simulink model "mohinh"  (R2017a)
settings: Solver=FixedStepDiscrete  StartTime=0.0  StopTime=5  RelTol=1e-3
undefined symbols (not defined in the file): ln
libraries: powerlib x16, electricdrivelib x2, simulink x1, re_lib x1
settings Model: Creator=huynh_000  LastModifiedBy=huynh_000

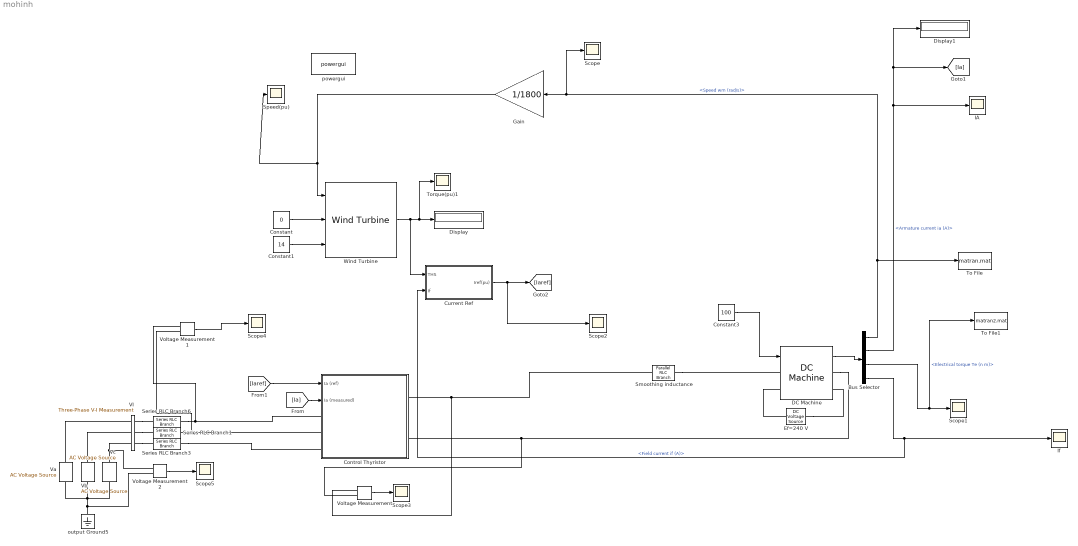
== system mohinh ==
  Bus Selector : BusSelector  OutputSignals=Speed wm (rad/s),Armature current ia (A),Electrical torque Te (n m),Field current if (A)
  Constant : Constant  Value=0
  Constant1 : Constant  Value=14
  Constant3 : Constant  Value=100
  Control Thyristor : Subsystem
  Current Ref : Subsystem
  DC Machine : powerlib/Machines/DC Machine  PresetModel=No  MechanicalLoad=Torque TL  FieldType=Wound  ShowDetailedParameters=on  MeasurementBus=off  RLa="[ 0.5  0.01]"  RLf="[240  120]"  Laf=1.8  MachineConstant=Torque constant (N.m/A)  Ke=1.8  Kt=1.8  J=2  Bm=0.5  Tf=0  w0=1  Ifinit=1  TsPowergui=0  TsBlock=-1
  Display : Display
  Display1 : Display
  Ef=240 V : powerlib/Electrical Sources/DC Voltage Source  Description=source block  Amplitude=240  Measurements=None
      settings: AttributesFormatString=\n
  Gain : Gain  Gain=1/1800
  IA : Scope
  If : Scope
  Scope{,1..5} (6 alike) : Scope
  Series RLC Branch1 : powerlib/Elements/Series RLC Branch  LConnTagsString=__new0  RConnTagsString=__new0  BranchType=RL  Resistance=0.01  Inductance=1e-3  SetiL0=off  InitialCurrent=0  Capacitance=[]  Setx0=off  InitialVoltage=0  Measurements=None
  Series RLC Branch3 : powerlib/Elements/Series RLC Branch  LConnTagsString=__new0  RConnTagsString=__new0  BranchType=RL  Resistance=0.01  Inductance=1e-3  SetiL0=off  InitialCurrent=0  Capacitance=[]  Setx0=off  InitialVoltage=0  Measurements=None
  Series RLC Branch6 : powerlib/Elements/Series RLC Branch  LConnTagsString=__new0  RConnTagsString=__new0  BranchType=RL  Resistance=0.01  Inductance=1e-3  SetiL0=off  InitialCurrent=0  Capacitance=[]  Setx0=off  InitialVoltage=0  Measurements=None
  Smoothing inductance : powerlib/Elements/Parallel RLC Branch  LConnTagsString=a  RConnTagsString=__new0  BranchType=L  Resistance=[]  Inductance=50e-3  SetiL0=off  InitialCurrent=0  Capacitance=[]  Setx0=off  InitialVoltage=0  Measurements=None
  Speed(pu) : Scope
  To File : ToFile  Filename=matran.mat  MatrixName=speed
  To File1 : ToFile  Filename=matran2.mat  MatrixName=torque
  Torque(pu)1 : Scope
  VI : powerlib/Measurements/Three-Phase V-I Measurement  VoltageMeasurement=phase-to-ground  SetLabelV=on  LabelV=Vabc  Vpu=on  VpuLL=off  CurrentMeasurement=yes  SetLabelI=on  LabelI=Iabc  Ipu=off  Pbase=100e6  Vbase=208  OutputType=Complex  PhasorSimulation=off  PSBequivalent=0
  Va : powerlib/Electrical Sources/AC Voltage Source  Description=source block  Amplitude=220*sqrt(2)  Phase=0  Frequency=60  SampleTime=0  Measurements=None  BusType=swing  Pref=10e3  Qref=0  Qmin=-inf  Qmax=+inf
      settings: AttributesFormatString=\n
  Vb : powerlib/Electrical Sources/AC Voltage Source  Description=source block  Amplitude=220*sqrt(2)  Phase=-120  Frequency=60  SampleTime=0  Measurements=None  BusType=swing  Pref=10e3  Qref=0  Qmin=-inf  Qmax=+inf
      settings: AttributesFormatString=\n
  Vc : powerlib/Electrical Sources/AC Voltage Source  Description=source block  Amplitude=220*sqrt(2)  Phase=120  Frequency=60  SampleTime=0  Measurements=None  BusType=swing  Pref=10e3  Qref=0  Qmin=-inf  Qmax=+inf
      settings: AttributesFormatString=\n
  Voltage Measurement : powerlib/Measurements/Voltage Measurement  PhasorSimulation=off  OutputType=Complex  PSBequivalent=0
  Voltage Measurement1 : powerlib/Measurements/Voltage Measurement  PhasorSimulation=off  OutputType=Complex  PSBequivalent=0
  Voltage Measurement2 : powerlib/Measurements/Voltage Measurement  PhasorSimulation=off  OutputType=Complex  PSBequivalent=0
  Wind Turbine : re_lib/Wind Generation/Wind Turbine  Pnom=20000  Pelec_base=20000/0.9  wind_base=12  P_wind_base=0.73  speed_nom=1.2  pitch_angle=0  c1_c6="[0.51763          116          0.4            5           21     0.006795]"  cp_nom=0.48  lambda_nom=8.1
      settings: SourceProductName=Simscape Power Systems  SourceProductBaseCode=PS
  output Ground5 : powerlib/Elements/Ground  LConnTagsString=a
  powergui : powerlib/powergui  Priority=1  SimulationMode=Discrete  SampleTime=0.001  frequency=60  Iterations=50  frequencyindice=0  Pbase=100e6  ErrMax=1e-4  UnitsV=kV  UnitsW=MW  buscounter=0  FunctionMessages=off  echomessages=off  EnableUseOfTLC=off  CurrentSourceSwitches=off  DisableSnubberDevices=off  DisableRonSwitches=off  DisableVfSwitches=off  DisplayEquations=off  SolverType=Tustin/Backward Euler (TBE)  Interpol=off  ExternalGateDelay=off  methode=off  Ts=100  x0status=blocks  SPID=on  SwTol=0  HookPort=off  RestoreLinks=warning  ResistiveCurrentMeasurement=off  Frange=[0:2:500]  Ylog=off  Xlog=on  ShowGrid=off  save=off  variable=ZData  structure=0  ZoomFFT=off  StartTime=0.0  cycles=1  DisplayStyle=1  fundamental=60  FreqAxis=off  MaxFrequency=1000  frequencyindicesteady=1  RmsSteady=1  display=off
  wires:
  Constant/1 -> Wind Turbine/2
  Constant1/1 -> Wind Turbine/3
  DC Machine/1 -> Bus Selector/1
  Bus Selector/1 -> To File/1, Scope/1, Gain/1  "<Speed wm (rad/s)>"
  Bus Selector/2 -> Display1/1, [Ia], IA/1  "<Armature current ia (A)>"
  [Ia] -> Control Thyristor/2("Ia (measured) ")
  Wind Turbine/1 -> Current Ref/1(THS), Torque(pu)1/1, Display/1
  Current Ref/1(Iref(pu)) -> Scope2/1, [Iaref]
  [Iaref] -> Control Thyristor/1("Ia (ref) ")
  Gain/1 -> Speed(pu)/1, Wind Turbine/1
  Bus Selector/3 -> To File1/1, Scope1/1  "<Electrical torque Te (n m)>"
  Bus Selector/4 -> Current Ref/2(If), If/1  "<Field current if (A)>"
  Voltage Measurement/1 -> Scope3/1
  Voltage Measurement1/1 -> Scope4/1
  Constant3/1 -> DC Machine/1
  Voltage Measurement2/1 -> Scope5/1
  connections:
  Series RLC Branch6/RConn1 -- Voltage Measurement1/LConn1 -- Control Thyristor/LConn1
  Smoothing inductance/RConn1 -- DC Machine/LConn1
  Smoothing inductance/LConn1 -- Voltage Measurement/LConn1 -- Control Thyristor/RConn1
  DC Machine/RConn1 -- Voltage Measurement/LConn2 -- Control Thyristor/RConn2
  Ef=240 V/RConn1 -- DC Machine/LConn2
  Ef=240 V/LConn1 -- DC Machine/RConn2
  Vb/LConn1 -- Voltage Measurement2/LConn2 -- output Ground5/LConn1 -- Vc/LConn1 -- Va/LConn1
  VI/RConn2 -- Series RLC Branch1/LConn1
  Vb/RConn1 -- VI/LConn2
  Va/RConn1 -- VI/LConn1
  VI/RConn3 -- Series RLC Branch3/LConn1
  Vc/RConn1 -- Voltage Measurement2/LConn1 -- VI/LConn3
  VI/RConn1 -- Series RLC Branch6/LConn1
  Series RLC Branch3/RConn1 -- Control Thyristor/LConn3
  Series RLC Branch1/RConn1 -- Voltage Measurement1/LConn2 -- Control Thyristor/LConn2

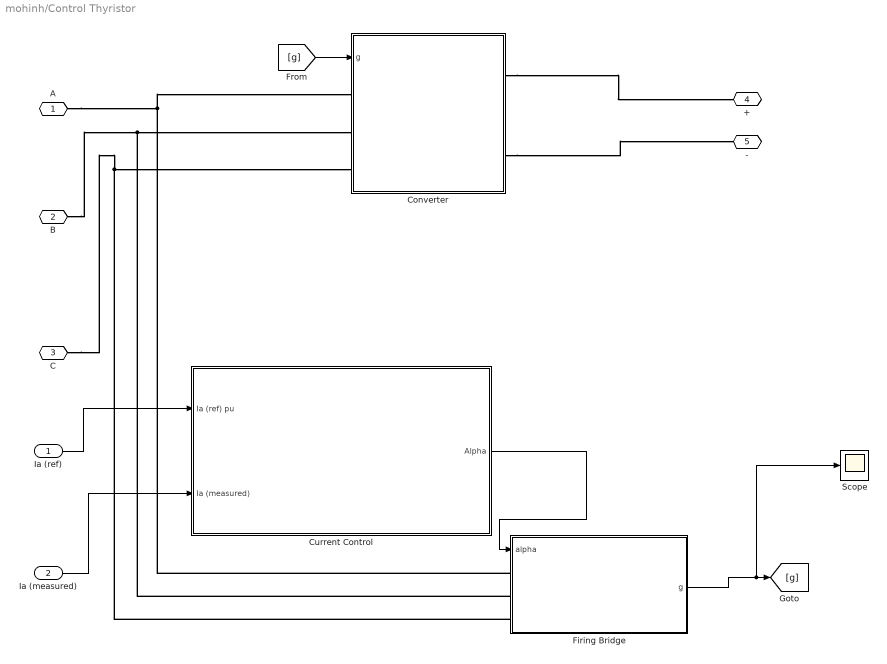
== system mohinh/Control Thyristor ==
  "Ia (ref) " : Inport
  "Ia (measured) " : Inport  Port=2
  Converter : Subsystem
  Current Control : Subsystem
  Firing Bridge : Subsystem
  Scope : Scope
  A : PMIOPort  Port=1  Side=Left
  B : PMIOPort  Port=2  Side=Left
  C : PMIOPort  Port=3  Side=Left
  + : PMIOPort  Tag=PMCPort  Port=4  Side=Right
  - : PMIOPort  Tag=PMCPort  Port=5  Side=Right
  wires:
  [g] -> Converter/1("g ")
  Firing Bridge/1("g ") -> Scope/1, [g]
  Current Control/1(" Alpha") -> Firing Bridge/1(alpha)
  "Ia (ref) "/1 -> Current Control/1(Ia (ref) pu)
  "Ia (measured) "/1 -> Current Control/2(Ia (measured))
  connections:
  A/RConn1 -- Firing Bridge/LConn1 -- Converter/LConn1
  B/RConn1 -- Firing Bridge/LConn2 -- Converter/LConn2
  C/RConn1 -- Firing Bridge/LConn3 -- Converter/LConn3
  Converter/RConn1 -- +/RConn1
  Converter/RConn2 -- -/RConn1

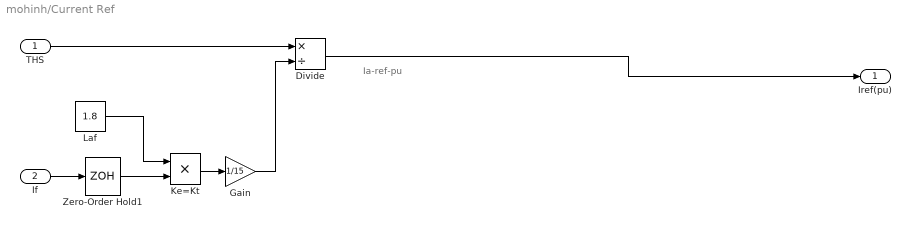
== system mohinh/Current Ref ==
  note: Ia-ref-pu
  THS : Inport
  If : Inport  Port=2
  Divide : Product  Inputs=*/
  Gain : Gain  Gain=1/15
  Ke=Kt : Product
  Laf : Constant  Value=1.8
  Zero-Order Hold1 : ZeroOrderHold  SampleTime=-1
  Iref(pu) : Outport
  wires:
  Laf/1 -> Ke=Kt/1
  THS/1 -> Divide/1
  If/1 -> Zero-Order Hold1/1
  Zero-Order Hold1/1 -> Ke=Kt/2
  Ke=Kt/1 -> Gain/1
  Gain/1 -> Divide/2
  Divide/1 -> Iref(pu)/1

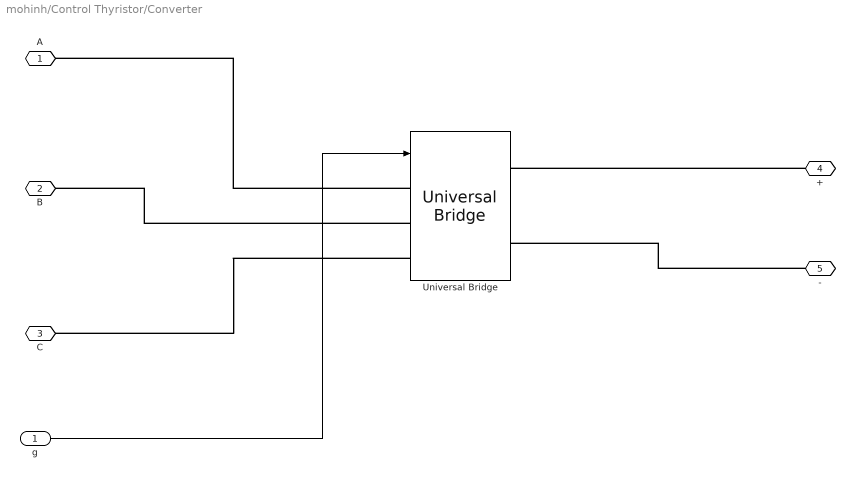
== system mohinh/Control Thyristor/Converter ==
  "g " : Inport
  Universal Bridge : powerlib/Power Electronics/Universal Bridge  Arms=3  SnubberResistance=1e5  SnubberCapacitance=inf  Device=Thyristors  Ron=1e-3  Lon=0  ForwardVoltages="[  0  0  ]"  ForwardVoltage=0  GTOparameters=[ 10e-6 , 20e-6 ]  IGBTparameters=[ 1e-6 , 2e-6 ]  Measurements=None  Measurements_2=None  converterType=Rectifier
  A : PMIOPort  Port=1  Side=Left
  B : PMIOPort  Port=2  Side=Left
  C : PMIOPort  Port=3  Side=Left
  + : PMIOPort  Tag=PMCPort  Port=4  Side=Right
  - : PMIOPort  Tag=PMCPort  Port=5  Side=Right
  wires:
  "g "/1 -> Universal Bridge/1
  connections:
  Universal Bridge/LConn1 -- A/RConn1
  Universal Bridge/LConn2 -- B/RConn1
  Universal Bridge/LConn3 -- C/RConn1
  +/RConn1 -- Universal Bridge/RConn1
  -/RConn1 -- Universal Bridge/RConn2

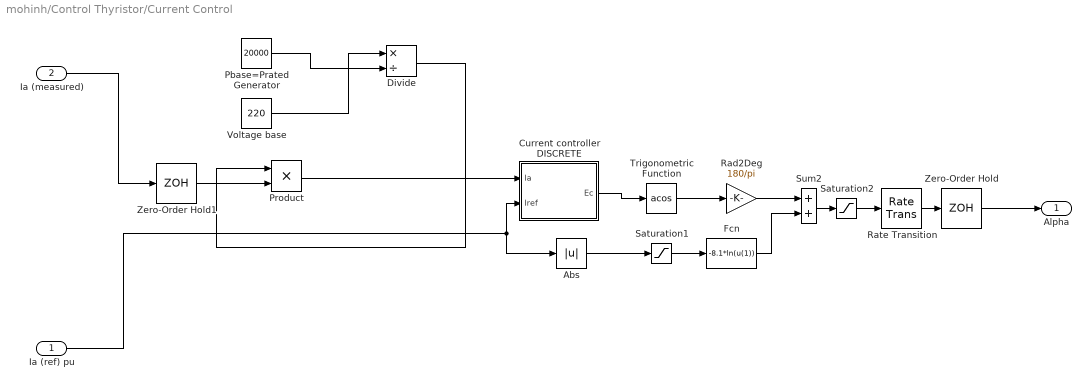
== system mohinh/Control Thyristor/Current Control ==
  Ia (ref) pu : Inport
  Ia (measured) : Inport  Port=2
  Abs : Abs  SaturateOnIntegerOverflow=on
  Current controller DISCRETE : Subsystem  AncestorBlock=|  mask(PI controller){Kp=1, Ki=80, Ts=100e-6}
      | electricdrivelib/Fundamental Drive Blocks/Current Controller
      | (DC)/current_controller/Rectifier_2q/Current controller
      | DISCRETE
      mask prompts: Kp "Proportional gain (Kp)"; Ki "Integral gain (Ki)"; Ts "Sample time (s) :"
      mask help: Proportional-Integral Speed Controller
      mask Display: plot(0,0,100,100,[35,35,65],[70,30,30],[35,65],[45,60])
  Divide : Product  Inputs=*/
  Fcn : Fcn  Expr=-8.1*ln(u(1))
  Pbase=Prated Generator : Constant  Value=20000
  Product : Product
  Rad2Deg : Gain  Gain=180/pi  SaturateOnIntegerOverflow=on  OutDataTypeStr=Inherit: Same as input  ParamDataTypeStr=Inherit: Same as input
  Rate Transition : RateTransition
  Saturation1 : Saturate  UpperLimit=1  LowerLimit=0.0005
  Saturation2 : Saturate  UpperLimit=160  LowerLimit=20
  Sum2 : Sum  SaturateOnIntegerOverflow=on  InputSameDT=on  OutDataTypeStr=Inherit: Same as first input
  Trigonometric Function : Trigonometry  Operator=acos
  Voltage base : Constant  Value=220
  Zero-Order Hold : ZeroOrderHold  SampleTime=100e-6
  Zero-Order Hold1 : ZeroOrderHold  SampleTime=100e-6
  " Alpha" : Outport
  wires:
  Saturation1/1 -> Fcn/1
  Abs/1 -> Saturation1/1
  Rad2Deg/1 -> Sum2/1
  Trigonometric Function/1 -> Rad2Deg/1
  Fcn/1 -> Sum2/2
  Ia (measured)/1 -> Zero-Order Hold1/1
  Zero-Order Hold/1 -> " Alpha"/1
  Saturation2/1 -> Rate Transition/1
  Product/1 -> Current controller DISCRETE/1(Ia)
  Ia (ref) pu/1 -> Current controller DISCRETE/2(Iref), Abs/1
  Current controller DISCRETE/1(Ec) -> Trigonometric Function/1
  Rate Transition/1 -> Zero-Order Hold/1
  Sum2/1 -> Saturation2/1
  Zero-Order Hold1/1 -> Product/2
  Voltage base/1 -> Divide/1
  Pbase=Prated Generator/1 -> Divide/2
  Divide/1 -> Product/1

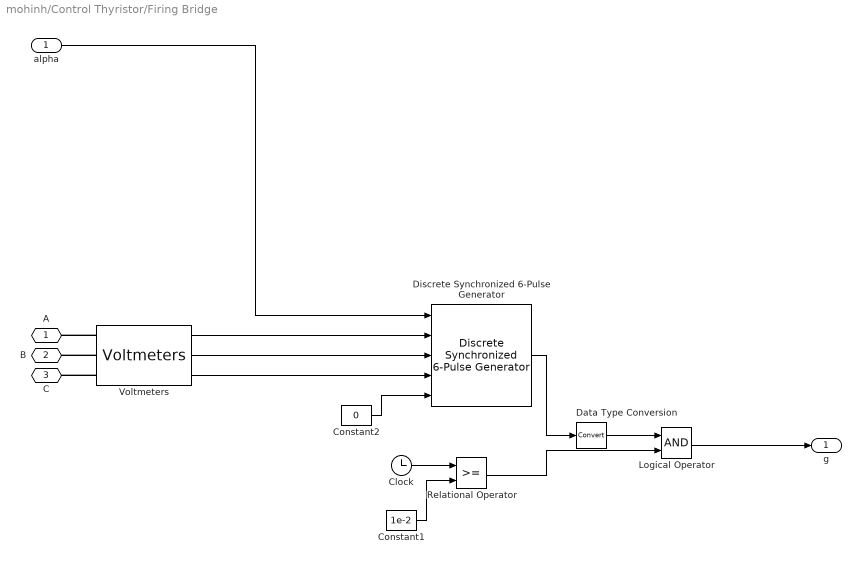
== system mohinh/Control Thyristor/Firing Bridge ==
  alpha : Inport
  Clock : Clock
  Constant1 : Constant  Value=1e-2
  Constant2 : Constant  Value=0
  Data Type Conversion : DataTypeConversion  SaturateOnIntegerOverflow=on  RndMeth=Zero
  Discrete Synchronized 6-Pulse Generator : electricdrivelib/Fundamental Drive Blocks/Bridge Firing Unit (DC)/Bridge firing unit/Detailed_3ph_2q/AC_Detailed_2q/Discrete Synchronized 6-Pulse Generator  freq=200  pwidth=180  Double_Pulse=on  Ts=100e-6
      settings: SourceProductName=Simscape Power Systems  SourceProductBaseCode=PS
  Logical Operator : Logic
  Relational Operator : RelationalOperator  RndMeth=Nearest  InputSameDT=on
  Voltmeters : electricdrivelib/Fundamental Drive Blocks/Bridge Firing Unit (DC)/Bridge firing unit/Detailed_3ph_2q/AC_Detailed_2q/Voltmeters
      settings: SourceProductName=Simscape Power Systems  SourceProductBaseCode=PS
  A : PMIOPort  Port=1  Side=Left
  B : PMIOPort  Port=2  Side=Left
  C : PMIOPort  Port=3  Side=Left
  "g " : Outport
  wires:
  Data Type Conversion/1 -> Logical Operator/1
  Voltmeters/3 -> Discrete Synchronized 6-Pulse Generator/4
  Clock/1 -> Relational Operator/1
  Logical Operator/1 -> "g "/1
  Constant2/1 -> Discrete Synchronized 6-Pulse Generator/5
  Voltmeters/2 -> Discrete Synchronized 6-Pulse Generator/3
  Constant1/1 -> Relational Operator/2
  Relational Operator/1 -> Logical Operator/2
  Discrete Synchronized 6-Pulse Generator/1 -> Data Type Conversion/1
  Voltmeters/1 -> Discrete Synchronized 6-Pulse Generator/2
  alpha/1 -> Discrete Synchronized 6-Pulse Generator/1
  connections:
  Voltmeters/LConn1 -- A/RConn1
  Voltmeters/LConn2 -- B/RConn1
  Voltmeters/LConn3 -- C/RConn1

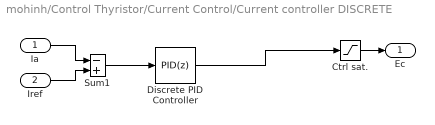
== system mohinh/Control Thyristor/Current Control/Current controller DISCRETE ==
  Ia : Inport
  Iref : Inport  Port=2
  Ctrl sat. : Saturate  UpperLimit=1  LowerLimit=-1
  Discrete PID Controller : simulink/Continuous/PID Controller  Controller=PID  TimeDomain=Discrete-time  SampleTime=-1  IntegratorMethod=Forward Euler  FilterMethod=Forward Euler  Form=Parallel  UseFilter=on  ControllerParametersSource=internal  P=1  I=80  D=0  N=100  InitialConditionSource=internal  InitialConditionForIntegrator=0  InitialConditionForFilter=0  ExternalReset=none  LimitOutput=off  UpperSaturationLimit=inf  LowerSaturationLimit=-inf  LinearizeAsGain=off  AntiWindupMode=none  Kb=1  TrackingMode=off  Kt=1  PParamMin=[]  PParamMax=[]  IParamMin=[]  IParamMax=[]  DParamMin=[]  DParamMax=[]  NParamMin=[]  NParamMax=[]  KbParamMin=[]  KbParamMax=[]  KtParamMin=[]  KtParamMax=[]  POutMin=[]  POutMax=[]  IOutMin=[]  IOutMax=[]  DOutMin=[]  DOutMax=[]  NOutMin=[]  NOutMax=[]  KbOutMin=[]  KbOutMax=[]  KtOutMin=[]  KtOutMax=[]  IntegratorOutMin=[]  IntegratorOutMax=[]  FilterOutMin=[]  FilterOutMax=[]  SumOutMin=[]  SumOutMax=[]  SumI1OutMin=[]  SumI1OutMax=[]  SumI2OutMin=[]  SumI2OutMax=[]  SumI3OutMin=[]  SumI3OutMax=[]  SumDOutMin=[]  SumDOutMax=[]  SaturationOutMin=[]  SaturationOutMax=[]  IntegratorContinuousStateAttributes=''  IntegratorStateMustResolveToSignalObject=off  IntegratorRTWStateStorageClass=Auto  FilterContinuousStateAttributes=''  FilterStateMustResolveToSignalObject=off  FilterRTWStateStorageClass=Auto  DifferentiatorICPrevScaledInput=0  DifferentiatorOutMin=[]  DifferentiatorOutMax=[]  InitialConditionSetting=State (most efficient)
  Sum1 : Sum  Inputs=-+  SaturateOnIntegerOverflow=on  InputSameDT=on  OutDataTypeStr=Inherit: Same as first input
  Ec : Outport  InitialOutput=0
  wires:
  Ia/1 -> Sum1/1
  Iref/1 -> Sum1/2
  Ctrl sat./1 -> Ec/1
  Sum1/1 -> Discrete PID Controller/1
  Discrete PID Controller/1 -> Ctrl sat./1
